simulink model "MotorControlLibNEWFixedP_FULL19b"  (R2020b)
settings: Solver=FixedStepDiscrete  StartTime=0.0  StopTime=100  FixedStep=Ts  RelTol=1e-3
values from neighbouring files (symbols this model uses):
  Ki_Iab_EMFobs = 1600.0    [MotorControl.sldd]
  Kp_Iab_EMFobs = 0.255    [MotorControl.sldd]
  p = 8/2    (= 4)    [MotorControlLibData.m]    (also in local_pmsm_torque_control_data.m = 8)
  Ts = 250.0e-06    (= 0.00025)    [MotorControlLibData.m]    (also in local_pmsm_torque_control_data.m = 5e-06)
undefined symbols (not defined in the file or in its folder): BrkPoints, CuttOffFreq_c, d_q_Voltage_Limiter_max, d_q_Voltage_Limiter_sat_neg, d_q_Voltage_Limiter_sat_pos, DiscIntNeverNeededParam, Down, dSoll, EMFobsLdGain, EMFobsRS, Ki_dAxis, Ki_qAxis, Kp_dAxis, Kp_qAxis, MaxBckEMFVol_sat_neg, MaxBckEMFVol_sat_pos, NumBits1, NumBits2, pwmTableData, qSoll, Slope1, Slope2, TqToIqConst, TsIntern, Up
libraries: simulink x13, pid_lib x6, eePwmGenerator x3, simulink_extras x2
(part 2 of 3)

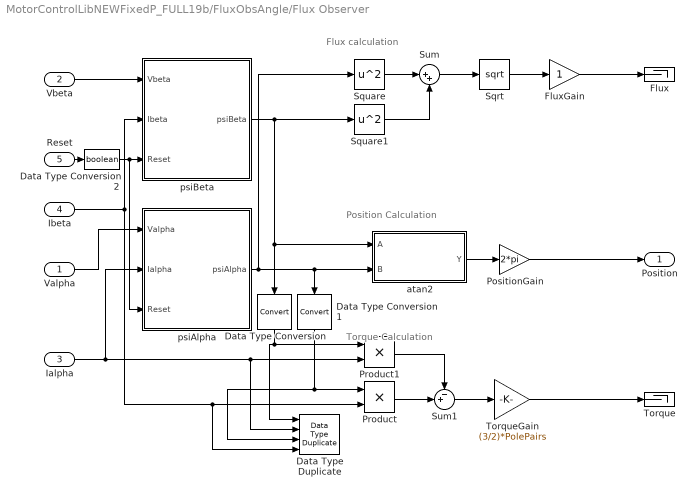
== system MotorControlLibNEWFixedP_FULL19b/FluxObsAngle/Flux Observer ==
  note: Torque Calculation
  note: Position Calculation
  note: Flux calculation
  Valpha : Inport  SampleTime=BlockSampleTime
  Vbeta : Inport  Port=2  SampleTime=BlockSampleTime
  Ialpha : Inport  Port=3  SampleTime=BlockSampleTime
  Ibeta : Inport  Port=4  SampleTime=BlockSampleTime
  Reset : Inport  Port=5  SampleTime=BlockSampleTime
  Data Type Duplicate : DataTypeDuplicate  NumInputPorts=4
  Data Type Conversion : DataTypeConversion  RndMeth=Simplest
  Data Type Conversion1 : DataTypeConversion  RndMeth=Simplest
  Data Type Conversion2 : DataTypeConversion  OutDataTypeStr=boolean  RndMeth=Simplest
  Flux : Terminator
  FluxGain : Gain  OutDataTypeStr=FluxDatatype  RndMeth=Simplest
  PositionGain : Gain  Gain=2*pi  OutDataTypeStr=PositionDatatype  RndMeth=Simplest
  Product : Product  RndMeth=Simplest  OutDataTypeStr=Inherit: Same as first input
  Product1 : Product  RndMeth=Simplest  OutDataTypeStr=Inherit: Same as first input
  Sqrt : Sqrt  RndMeth=Simplest  IntermediateResultsDataTypeStr=Inherit: Inherit from input  SaturateOnIntegerOverflow=on
  Square : Math  Operator=square  RndMeth=Simplest  SaturateOnIntegerOverflow=on
  Square1 : Math  Operator=square  RndMeth=Simplest  SaturateOnIntegerOverflow=on
  Sum : Sum  Inputs=|++
  Sum1 : Sum  Inputs=-+|
  Torque : Terminator
  TorqueGain : Gain  Gain=(3/2)*PolePairs  OutDataTypeStr=TorqueDatatype
  atan2 : Subsystem  TreatAsAtomicUnit=on  mask(atan2){outputUnit=PerUnit}
      mask prompts: outputUnit "Output unit:"
      mask help:
      | Compute the four-quadrant arctangent for two real numbers.
      |
      | The output datatype is identical to the inputs.
      |
      | The block output ranges from -pi to +pi (Radians) or 0 to 1 (PerUnit).
      mask Help: eval('mcb.internal.helpview(''atantwo'')')
      mask TypeOptions outputUnit: Radians | PerUnit
      mask Callback outputUnit: set_param([gcb, '/a16'],'AlgorithmParameterValue1',get_param(gcb,'outputUnit'))
      mask DialogControl Container7 Prompt: Parameters
      mask Display:
      | color('black');
      | port_label('input',1, 'A');
      | port_label('input',2, 'B');,
      | port_label('output',1, '\theta', 'interpreter', 'tex');
      | fprintf('atan2');
  psiAlpha : Subsystem
  psiBeta : Subsystem
  Position : Outport
  wires:
  Valpha/1 -> psiAlpha/1(Valpha)
  Ibeta/1 -> psiBeta/2(Ibeta), Data Type Duplicate/4, Product/2
  Vbeta/1 -> psiBeta/1(Vbeta)
  Reset/1 -> Data Type Conversion2/1
  TorqueGain/1 -> Torque/1
  Product/1 -> Sum1/2
  psiBeta/1(psiBeta) -> Square1/1, atan2/1(A), Data Type Conversion/1
  psiAlpha/1(psiAlpha) -> atan2/2(B), Data Type Conversion1/1, Square/1
  Ialpha/1 -> psiAlpha/2(Ialpha), Data Type Duplicate/2, Product1/2
  Product1/1 -> Sum1/1
  Sum1/1 -> TorqueGain/1
  FluxGain/1 -> Flux/1
  Square/1 -> Sum/1
  Sum/1 -> Sqrt/1
  Square1/1 -> Sum/2
  Sqrt/1 -> FluxGain/1
  PositionGain/1 -> Position/1
  atan2/1(Y) -> PositionGain/1
  Data Type Conversion/1 -> Data Type Duplicate/1, Product1/1
  Data Type Conversion1/1 -> Data Type Duplicate/3, Product/1
  Data Type Conversion2/1 -> psiAlpha/3(Reset), psiBeta/3(Reset)

== system MotorControlLibNEWFixedP_FULL19b/Inverse Park Transform/Switch_Axis ==
  A : Inport
  B : Inport  Port=2
  D_axis_aligned : Mux  Inputs=2
  Demux : Demux  Outputs=2
  Offset : Constant  Value=0  OutDataTypeStr=uint16  SampleTime=-1
  Q_axis_aligned : Mux  Inputs=2
  Switch : Switch  Criteria=u2 > Threshold  Threshold=1  RndMeth=Simplest  ZeroCross=off
  Unary_Minus : UnaryMinus
  Alpha : Outport  VectorParamsAs1DForOutWhenUnconnected=off
  Beta : Outport  Port=2  VectorParamsAs1DForOutWhenUnconnected=off
  wires:
  A/1 -> D_axis_aligned/1, Unary_Minus/1
  Unary_Minus/1 -> Q_axis_aligned/2
  Demux/2 -> Beta/1
  Switch/1 -> Demux/1
  B/1 -> D_axis_aligned/2, Q_axis_aligned/1
  Demux/1 -> Alpha/1
  Offset/1 -> Switch/2
  Q_axis_aligned/1 -> Switch/1
  D_axis_aligned/1 -> Switch/3

== system MotorControlLibNEWFixedP_FULL19b/PI_Controller/disable integrator on start up ==
  Add2 : Sum
  Compare To Constant : simulink/Logic and Bit Operations/Compare To Constant  relop=<  const=1500  OutDataTypeStr=boolean
  Constant8 : Constant  OutDataTypeStr=uint8
  Unit Delay : UnitDelay  SampleTime=-1  HasFrameUpgradeWarning=on
  time out : Outport
  wires:
  Add2/1 -> Unit Delay/1, Compare To Constant/1
  Constant8/1 -> Add2/1
  Compare To Constant/1 -> time out/1
  Unit Delay/1 -> Add2/2

== system MotorControlLibNEWFixedP_FULL19b/PWM Output/Inverse Clarke Transform ==
  In1 : Inport
  In2 : Inport  Port=2
  Data Type Duplicate : DataTypeDuplicate
  add_b : Sum  Inputs=-+  RndMeth=Simplest  OutDataTypeStr=Inherit: Same as first input
  add_c : Sum  Inputs=--  RndMeth=Simplest  OutDataTypeStr=Inherit: Same as first input
  one_by_two : Gain  Gain=1/2  RndMeth=Simplest  OutDataTypeStr=Inherit: Same as input
  sqrt3_by_two : Gain  Gain=sqrt(3)/2  RndMeth=Simplest  OutDataTypeStr=Inherit: Same as input
  a : Outport  VectorParamsAs1DForOutWhenUnconnected=off
  b : Outport  Port=2  VectorParamsAs1DForOutWhenUnconnected=off
  c : Outport  Port=3  VectorParamsAs1DForOutWhenUnconnected=off
  wires:
  add_c/1 -> c/1
  sqrt3_by_two/1 -> add_c/2, add_b/2
  In1/1 -> one_by_two/1, Data Type Duplicate/1, a/1
  one_by_two/1 -> add_b/1, add_c/1
  In2/1 -> sqrt3_by_two/1, Data Type Duplicate/2
  add_b/1 -> b/1

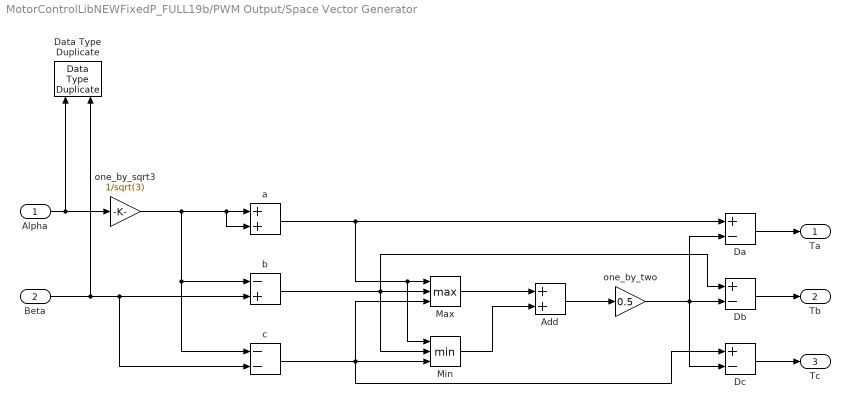
== system MotorControlLibNEWFixedP_FULL19b/PWM Output/Space Vector Generator ==
  Alpha : Inport
  Beta : Inport  Port=2
  Add : Sum  RndMeth=Simplest  OutDataTypeStr=Inherit: Same as first input
  Da : Sum  Inputs=+-  RndMeth=Simplest  OutDataTypeStr=Inherit: Same as first input
  Data Type Duplicate : DataTypeDuplicate
  Db : Sum  Inputs=+-  RndMeth=Simplest  OutDataTypeStr=Inherit: Same as first input
  Dc : Sum  Inputs=+-  RndMeth=Simplest  OutDataTypeStr=Inherit: Same as first input
  Max : MinMax  Function=max  Inputs=3  RndMeth=Simplest
  Min : MinMax  Inputs=3  RndMeth=Simplest
  a : Sum  RndMeth=Simplest  OutDataTypeStr=Inherit: Same as first input
  b : Sum  Inputs=-+  RndMeth=Simplest  OutDataTypeStr=Inherit: Same as first input
  c : Sum  Inputs=--  RndMeth=Simplest  OutDataTypeStr=Inherit: Same as first input
  one_by_sqrt3 : Gain  Gain=1/sqrt(3)  RndMeth=Simplest  OutDataTypeStr=Inherit: Same as input  ParamDataTypeStr=Inherit: Same as input
  one_by_two : Gain  Gain=0.5  RndMeth=Simplest  OutDataTypeStr=Inherit: Same as input  ParamDataTypeStr=Inherit: Same as input
  Ta : Outport  VectorParamsAs1DForOutWhenUnconnected=off
  Tb : Outport  Port=2  VectorParamsAs1DForOutWhenUnconnected=off
  Tc : Outport  Port=3  VectorParamsAs1DForOutWhenUnconnected=off
  wires:
  Db/1 -> Tb/1
  Dc/1 -> Tc/1
  Da/1 -> Ta/1
  a/1 -> Max/1, Min/1, Da/1
  Max/1 -> Add/1
  one_by_two/1 -> Da/2, Db/2, Dc/2
  Add/1 -> one_by_two/1
  Min/1 -> Add/2
  Alpha/1 -> Data Type Duplicate/1, one_by_sqrt3/1
  one_by_sqrt3/1 -> a/1, a/2, b/1, c/1
  Beta/1 -> c/2, b/2, Data Type Duplicate/2
  b/1 -> Max/2, Min/2, Db/1
  c/1 -> Min/3, Dc/1, Max/3

== system MotorControlLibNEWFixedP_FULL19b/Park Transform/Switch_Axis ==
  d : Inport
  q : Inport  Port=2
  D_axis_aligned : Mux  Inputs=2
  Demux : Demux  Outputs=2
  Offset : Constant  Value=0  OutDataTypeStr=uint16  SampleTime=-1
  Q_axis_aligned : Mux  Inputs=2
  Switch : Switch  Criteria=u2 > Threshold  Threshold=1  RndMeth=Simplest  ZeroCross=off
  Unary_Minus : UnaryMinus
  d_axis : Outport  VectorParamsAs1DForOutWhenUnconnected=off
  q_axis : Outport  Port=2  VectorParamsAs1DForOutWhenUnconnected=off
  wires:
  D_axis_aligned/1 -> Switch/3
  Q_axis_aligned/1 -> Switch/1
  d/1 -> D_axis_aligned/1, Q_axis_aligned/2
  Offset/1 -> Switch/2
  Demux/1 -> d_axis/1
  Unary_Minus/1 -> Q_axis_aligned/1
  q/1 -> D_axis_aligned/2, Unary_Minus/1
  Switch/1 -> Demux/1
  Demux/2 -> q_axis/1

== system MotorControlLibNEWFixedP_FULL19b/Position observer/Atan2 ==
  In1 : Inport
  In2 : Inport  Port=2
  Atan2 : Trigonometry  Operator=atan2  ApproximationMethod=CORDIC  NumberOfIterations=6
  Data Type Conversion5 : DataTypeConversion
  Data Type Conversion6 : DataTypeConversion  OutDataTypeStr=single
  Data Type Conversion7 : DataTypeConversion  OutDataTypeStr=single
  Out1 : Outport
  wires:
  Atan2/1 -> Data Type Conversion5/1
  In1/1 -> Data Type Conversion6/1
  Data Type Conversion6/1 -> Atan2/1
  Data Type Conversion7/1 -> Atan2/2
  In2/1 -> Data Type Conversion7/1
  Data Type Conversion5/1 -> Out1/1

== system MotorControlLibNEWFixedP_FULL19b/Position observer/EMF Observer Ia ==
  Iab : Inport
  Vab : Inport  Port=2
  filtered emf : Inport  Port=3
  reset : Inport  Port=4
  Add6 : Sum  Inputs=-+  InputSameDT=on
  DC Motor Model : Subsystem  TreatAsAtomicUnit=on  SystemSampleTime=Ts
  PI Controller : Subsystem
  Rate Transition{,1..3} (4 alike) : RateTransition  Integrity=off
  Unit Delay : UnitDelay  SampleTime=-1  HasFrameUpgradeWarning=on
  BackEMFest : Outport
  wires:
  Iab/1 -> Add6/1
  DC Motor Model/1(i_integrated_en8) -> Rate Transition/1
  Vab/1 -> Rate Transition1/1
  Rate Transition/1 -> Add6/2  "Iest"
  Rate Transition1/1 -> DC Motor Model/2(In2)
  Rate Transition2/1 -> DC Motor Model/1(Sig_Emfobs_PI_out)
  PI Controller/1(Sig_Emfobs_PI_out) -> Unit Delay/1, BackEMFest/1  "BackEMF est"
  Add6/1 -> PI Controller/1(Sig_Emfobs_errorSum_m)  "Sig_Emfobs_errorSum_m"
  filtered emf/1 -> Rate Transition3/1
  Rate Transition3/1 -> DC Motor Model/3(In3)
  Unit Delay/1 -> Rate Transition2/1
  reset/1 -> PI Controller/2(reset)

== system MotorControlLibNEWFixedP_FULL19b/Position observer/EMF Observer Ia1 ==
  Iab : Inport
  Vab : Inport  Port=2
  DC Motor Model : Subsystem
  PI Controller : Subsystem
  Rate Transition : RateTransition
  Rate Transition1 : RateTransition
  Rate Transition2 : RateTransition
  Unit Delay : UnitDelay  SampleTime=-1  HasFrameUpgradeWarning=on
  Iestimated : Outport
  IestNEW : Outport  Port=2
  wires:
  DC Motor Model/1(Out1) -> Rate Transition/1
  Vab/1 -> Rate Transition1/1
  Rate Transition/1 -> PI Controller/2(In2), IestNEW/1
  Rate Transition1/1 -> DC Motor Model/2(In2)
  Rate Transition2/1 -> DC Motor Model/1(In1)
  PI Controller/1(Out1) -> Iestimated/1, Unit Delay/1
  Iab/1 -> PI Controller/1(In1)
  Unit Delay/1 -> Rate Transition2/1

== system MotorControlLibNEWFixedP_FULL19b/Position observer/EMF Observer Ia2 ==
  Iab : Inport
  Vab : Inport  Port=2
  filtered emf : Inport  Port=3
  reset : Inport  Port=4
  Add6 : Sum  Inputs=-+  InputSameDT=on
  DC Motor Model : Subsystem  TreatAsAtomicUnit=on  SystemSampleTime=Ts
  Data Type Conversion : DataTypeConversion
  PI Controller : Subsystem  TreatAsAtomicUnit=on
  Rate Transition{,1..3} (4 alike) : RateTransition  Integrity=off
  Unit Delay : UnitDelay  SampleTime=-1  HasFrameUpgradeWarning=on
  BackEMFest : Outport
  wires:
  PI Controller/1(Sig_Emfobs_PI_out) -> Unit Delay/1, BackEMFest/1
  Add6/1 -> PI Controller/1(Sig_Emfobs_errorSum_m)
  Rate Transition2/1 -> DC Motor Model/1(Sig_Emfobs_PI_out)
  Rate Transition1/1 -> DC Motor Model/2(In2)
  Rate Transition/1 -> Add6/2
  Vab/1 -> Rate Transition1/1
  DC Motor Model/1(i_integrated_en8) -> Rate Transition/1
  Iab/1 -> Data Type Conversion/1
  Data Type Conversion/1 -> Add6/1
  filtered emf/1 -> Rate Transition3/1
  Rate Transition3/1 -> DC Motor Model/3(Sig_Emfobs_PI_out1)
  Unit Delay/1 -> Rate Transition2/1
  reset/1 -> PI Controller/2(reset)

== system MotorControlLibNEWFixedP_FULL19b/Position observer/Low pass filter ==
  note: Integrator
  note: d/dt(i)
  In1 : Inport
  Add2 : Sum  Inputs=+-
  Constant : Constant  Value=Value  OutDataTypeStr=uint16
  Delay : Delay  DelayLength=1  InitialCondition=0
  Gain : Gain  Gain=Gain  ParamDataTypeStr=fixdt(1,16,2^-16,0)  OutDataTypeStr=fixdt(1,16,2^-14,0)  SaturateOnIntegerOverflow=on
  Product1 : Product  OutDataTypeStr=fixdt(1,16,2^-6,0)
  Sum : Sum  Inputs=|++  OutDataTypeStr=Inherit: Same as first input
  Unit Delay : UnitDelay  SampleTime=-1  HasFrameUpgradeWarning=on
  Output : Outport
  wires:
  Constant/1 -> Product1/2
  In1/1 -> Add2/1
  Add2/1 -> Gain/1
  Product1/1 -> Output/1, Unit Delay/1
  Gain/1 -> Sum/1
  Delay/1 -> Sum/2
  Sum/1 -> Delay/1, Product1/1
  Unit Delay/1 -> Add2/2

== system MotorControlLibNEWFixedP_FULL19b/Position observer/Low pass filter1 ==
  note: d/dt(i)
  note: Integrator
  In1 : Inport
  Add2 : Sum  Inputs=+-
  Constant : Constant  Value=Value  OutDataTypeStr=uint16
  Delay : Delay  DelayLength=1  InitialCondition=0
  Gain : Gain  Gain=Gain  ParamDataTypeStr=fixdt(1,16,2^-16,0)  OutDataTypeStr=fixdt(1,16,2^-14,0)  SaturateOnIntegerOverflow=on
  Product1 : Product  OutDataTypeStr=fixdt(1,16,2^-6,0)
  Sum : Sum  Inputs=|++  OutDataTypeStr=Inherit: Same as first input
  Unit Delay : UnitDelay  SampleTime=-1  HasFrameUpgradeWarning=on
  Output : Outport
  wires:
  Unit Delay/1 -> Add2/2
  Sum/1 -> Product1/1, Delay/1
  Delay/1 -> Sum/2
  Gain/1 -> Sum/1
  Product1/1 -> Unit Delay/1, Output/1
  Add2/1 -> Gain/1
  In1/1 -> Add2/1
  Constant/1 -> Product1/2

== system MotorControlLibNEWFixedP_FULL19b/Position observer/Low pass filter2 ==
  note: Integrator
  note: d/dt(i)
  In1 : Inport
  Add2 : Sum  Inputs=+-
  Constant : Constant  Value=Value  OutDataTypeStr=uint16
  Delay : Delay  DelayLength=1  InitialCondition=0
  Gain : Gain  Gain=Gain  ParamDataTypeStr=fixdt(1,16,2^-16,0)  OutDataTypeStr=fixdt(1,16,2^-14,0)  SaturateOnIntegerOverflow=on
  Product1 : Product  OutDataTypeStr=fixdt(1,16,2^-6,0)
  Sum : Sum  Inputs=|++  OutDataTypeStr=Inherit: Same as first input
  Unit Delay : UnitDelay  SampleTime=-1  HasFrameUpgradeWarning=on
  Output : Outport
  wires:
  Constant/1 -> Product1/2
  In1/1 -> Add2/1
  Add2/1 -> Gain/1
  Product1/1 -> Output/1, Unit Delay/1
  Gain/1 -> Sum/1
  Delay/1 -> Sum/2
  Sum/1 -> Delay/1, Product1/1
  Unit Delay/1 -> Add2/2

== system MotorControlLibNEWFixedP_FULL19b/Position observer/Low pass filter3 ==
  note: d/dt(i)
  note: Integrator
  In1 : Inport
  Add2 : Sum  Inputs=+-
  Constant : Constant  Value=Value  OutDataTypeStr=uint16
  Delay : Delay  DelayLength=1  InitialCondition=0
  Gain : Gain  Gain=Gain  ParamDataTypeStr=fixdt(1,16,2^-16,0)  OutDataTypeStr=fixdt(1,16,2^-14,0)  SaturateOnIntegerOverflow=on
  Product1 : Product  OutDataTypeStr=fixdt(1,16,2^-6,0)
  Sum : Sum  Inputs=|++  OutDataTypeStr=Inherit: Same as first input
  Unit Delay : UnitDelay  SampleTime=-1  HasFrameUpgradeWarning=on
  Output : Outport
  wires:
  Unit Delay/1 -> Add2/2
  Sum/1 -> Product1/1, Delay/1
  Delay/1 -> Sum/2
  Gain/1 -> Sum/1
  Product1/1 -> Unit Delay/1, Output/1
  Add2/1 -> Gain/1
  In1/1 -> Add2/1
  Constant/1 -> Product1/2

== system MotorControlLibNEWFixedP_FULL19b/Position observer fixed point/Atan2 ==
  In1 : Inport
  In2 : Inport  Port=2
  Atan2 : Trigonometry  Operator=atan2  ApproximationMethod=CORDIC  NumberOfIterations=6
  Data Type Conversion5 : DataTypeConversion
  Data Type Conversion6 : DataTypeConversion  OutDataTypeStr=single
  Data Type Conversion7 : DataTypeConversion  OutDataTypeStr=single
  Out1 : Outport
  wires:
  Atan2/1 -> Data Type Conversion5/1
  In1/1 -> Data Type Conversion6/1
  Data Type Conversion6/1 -> Atan2/1
  Data Type Conversion7/1 -> Atan2/2
  In2/1 -> Data Type Conversion7/1
  Data Type Conversion5/1 -> Out1/1

== system MotorControlLibNEWFixedP_FULL19b/Position observer fixed point/EMF Observer Ia ==
  Iab : Inport
  Vab : Inport  Port=2
  filtered emf : Inport  Port=3
  reset : Inport  Port=4
  Add6 : Sum  Inputs=-+  InputSameDT=on
  DC Motor Model : Subsystem  TreatAsAtomicUnit=on  SystemSampleTime=Ts
  PI Controller : Subsystem
  Rate Transition{,1..3} (4 alike) : RateTransition  Integrity=off
  Unit Delay : UnitDelay  SampleTime=-1  HasFrameUpgradeWarning=on
  BackEMFest : Outport
  wires:
  Iab/1 -> Add6/1
  DC Motor Model/1(i_integrated_en8) -> Rate Transition/1
  Vab/1 -> Rate Transition1/1
  Rate Transition/1 -> Add6/2  "Iest"
  Rate Transition1/1 -> DC Motor Model/2(In2)
  Rate Transition2/1 -> DC Motor Model/1(Sig_Emfobs_PI_out)
  PI Controller/1(Sig_Emfobs_PI_out) -> Unit Delay/1, BackEMFest/1  "BackEMF est"
  Add6/1 -> PI Controller/1(Sig_Emfobs_errorSum_m)  "Sig_Emfobs_errorSum_m"
  filtered emf/1 -> Rate Transition3/1
  Rate Transition3/1 -> DC Motor Model/3(In3)
  Unit Delay/1 -> Rate Transition2/1
  reset/1 -> PI Controller/2(reset)

== system MotorControlLibNEWFixedP_FULL19b/Position observer fixed point/EMF Observer Ia1 ==
  Iab : Inport
  Vab : Inport  Port=2
  DC Motor Model : Subsystem
  PI Controller : Subsystem
  Rate Transition : RateTransition
  Rate Transition1 : RateTransition
  Rate Transition2 : RateTransition
  Unit Delay : UnitDelay  SampleTime=-1  HasFrameUpgradeWarning=on
  Iestimated : Outport
  IestNEW : Outport  Port=2
  wires:
  DC Motor Model/1(Out1) -> Rate Transition/1
  Vab/1 -> Rate Transition1/1
  Rate Transition/1 -> PI Controller/2(In2), IestNEW/1
  Rate Transition1/1 -> DC Motor Model/2(In2)
  Rate Transition2/1 -> DC Motor Model/1(In1)
  PI Controller/1(Out1) -> Iestimated/1, Unit Delay/1
  Iab/1 -> PI Controller/1(In1)
  Unit Delay/1 -> Rate Transition2/1

== system MotorControlLibNEWFixedP_FULL19b/Position observer fixed point/EMF Observer Ia2 ==
  Iab : Inport
  Vab : Inport  Port=2
  filtered emf : Inport  Port=3
  reset : Inport  Port=4
  Add6 : Sum  Inputs=-+  InputSameDT=on
  DC Motor Model : Subsystem  TreatAsAtomicUnit=on  SystemSampleTime=Ts
  Data Type Conversion : DataTypeConversion
  PI Controller : Subsystem  TreatAsAtomicUnit=on
  Rate Transition{,1..3} (4 alike) : RateTransition  Integrity=off
  Unit Delay : UnitDelay  SampleTime=-1  HasFrameUpgradeWarning=on
  BackEMFest : Outport
  wires:
  PI Controller/1(Sig_Emfobs_PI_out) -> Unit Delay/1, BackEMFest/1
  Add6/1 -> PI Controller/1(Sig_Emfobs_errorSum_m)
  Rate Transition2/1 -> DC Motor Model/1(Sig_Emfobs_PI_out)
  Rate Transition1/1 -> DC Motor Model/2(In2)
  Rate Transition/1 -> Add6/2
  Vab/1 -> Rate Transition1/1
  DC Motor Model/1(i_integrated_en8) -> Rate Transition/1
  Iab/1 -> Data Type Conversion/1
  Data Type Conversion/1 -> Add6/1
  filtered emf/1 -> Rate Transition3/1
  Rate Transition3/1 -> DC Motor Model/3(Sig_Emfobs_PI_out1)
  Unit Delay/1 -> Rate Transition2/1
  reset/1 -> PI Controller/2(reset)

== system MotorControlLibNEWFixedP_FULL19b/Position observer fixed point/Low pass filter ==
  note: Integrator
  note: d/dt(i)
  In1 : Inport
  Add2 : Sum  Inputs=+-
  Constant : Constant  Value=Value  OutDataTypeStr=uint16
  Delay : Delay  DelayLength=1  InitialCondition=0
  Gain : Gain  Gain=Gain  ParamDataTypeStr=fixdt(1,16,2^-16,0)  OutDataTypeStr=fixdt(1,16,2^-14,0)  SaturateOnIntegerOverflow=on
  Product1 : Product  OutDataTypeStr=fixdt(1,16,2^-6,0)
  Sum : Sum  Inputs=|++  OutDataTypeStr=Inherit: Same as first input
  Unit Delay : UnitDelay  SampleTime=-1  HasFrameUpgradeWarning=on
  Output : Outport
  wires:
  Constant/1 -> Product1/2
  In1/1 -> Add2/1
  Add2/1 -> Gain/1
  Product1/1 -> Output/1, Unit Delay/1
  Gain/1 -> Sum/1
  Delay/1 -> Sum/2
  Sum/1 -> Delay/1, Product1/1
  Unit Delay/1 -> Add2/2

== system MotorControlLibNEWFixedP_FULL19b/Position observer fixed point/Low pass filter1 ==
  note: d/dt(i)
  note: Integrator
  In1 : Inport
  Add2 : Sum  Inputs=+-
  Constant : Constant  Value=Value  OutDataTypeStr=uint16
  Delay : Delay  DelayLength=1  InitialCondition=0
  Gain : Gain  Gain=Gain  ParamDataTypeStr=fixdt(1,16,2^-16,0)  OutDataTypeStr=fixdt(1,16,2^-14,0)  SaturateOnIntegerOverflow=on
  Product1 : Product  OutDataTypeStr=fixdt(1,16,2^-6,0)
  Sum : Sum  Inputs=|++  OutDataTypeStr=Inherit: Same as first input
  Unit Delay : UnitDelay  SampleTime=-1  HasFrameUpgradeWarning=on
  Output : Outport
  wires:
  Unit Delay/1 -> Add2/2
  Sum/1 -> Product1/1, Delay/1
  Delay/1 -> Sum/2
  Gain/1 -> Sum/1
  Product1/1 -> Unit Delay/1, Output/1
  Add2/1 -> Gain/1
  In1/1 -> Add2/1
  Constant/1 -> Product1/2

== system MotorControlLibNEWFixedP_FULL19b/Position observer fixed point/Low pass filter2 ==
  note: Integrator
  note: d/dt(i)
  In1 : Inport
  Add2 : Sum  Inputs=+-
  Constant : Constant  Value=Value  OutDataTypeStr=uint16
  Delay : Delay  DelayLength=1  InitialCondition=0
  Gain : Gain  Gain=Gain  ParamDataTypeStr=fixdt(1,16,2^-16,0)  OutDataTypeStr=fixdt(1,16,2^-14,0)  SaturateOnIntegerOverflow=on
  Product1 : Product  OutDataTypeStr=fixdt(1,16,2^-6,0)
  Sum : Sum  Inputs=|++  OutDataTypeStr=Inherit: Same as first input
  Unit Delay : UnitDelay  SampleTime=-1  HasFrameUpgradeWarning=on
  Output : Outport
  wires:
  Constant/1 -> Product1/2
  In1/1 -> Add2/1
  Add2/1 -> Gain/1
  Product1/1 -> Output/1, Unit Delay/1
  Gain/1 -> Sum/1
  Delay/1 -> Sum/2
  Sum/1 -> Delay/1, Product1/1
  Unit Delay/1 -> Add2/2

== system MotorControlLibNEWFixedP_FULL19b/Position observer fixed point/Low pass filter3 ==
  note: d/dt(i)
  note: Integrator
  In1 : Inport
  Add2 : Sum  Inputs=+-
  Constant : Constant  Value=Value  OutDataTypeStr=uint16
  Delay : Delay  DelayLength=1  InitialCondition=0
  Gain : Gain  Gain=Gain  ParamDataTypeStr=fixdt(1,16,2^-16,0)  OutDataTypeStr=fixdt(1,16,2^-14,0)  SaturateOnIntegerOverflow=on
  Product1 : Product  OutDataTypeStr=fixdt(1,16,2^-6,0)
  Sum : Sum  Inputs=|++  OutDataTypeStr=Inherit: Same as first input
  Unit Delay : UnitDelay  SampleTime=-1  HasFrameUpgradeWarning=on
  Output : Outport
  wires:
  Unit Delay/1 -> Add2/2
  Sum/1 -> Product1/1, Delay/1
  Delay/1 -> Sum/2
  Gain/1 -> Sum/1
  Product1/1 -> Unit Delay/1, Output/1
  Add2/1 -> Gain/1
  In1/1 -> Add2/1
  Constant/1 -> Product1/2

== system MotorControlLibNEWFixedP_FULL19b/Start up/Logic after motor is stoped ==
  In1 : Inport
  Compare To Zero : simulink/Logic and Bit Operations/Compare To Zero  relop===  OutDataTypeStr=boolean
  Detect Decrease : simulink/Logic and Bit Operations/Detect Decrease  vinit=0  OutDataTypeStr=boolean
  Enabled Subsystem : Subsystem  TreatAsAtomicUnit=on
  Enabled Subsystem1 : Subsystem  TreatAsAtomicUnit=on
  S-R Flip-Flop : simulink_extras/Flip Flops/S-R Flip-Flop  initial_condition=0
  S-R Flip-Flop1 : simulink_extras/Flip Flops/S-R Flip-Flop  initial_condition=0
  Terminator : Terminator
  Terminator1 : Terminator
  Unit Delay : UnitDelay  SampleTime=-1  HasFrameUpgradeWarning=on
  Unit Delay1 : UnitDelay  SampleTime=-1  HasFrameUpgradeWarning=on
  Out1 : Outport
  wires:
  Enabled Subsystem/1(Out1) -> S-R Flip-Flop1/1
  In1/1 -> Enabled Subsystem/1(In1), Compare To Zero/1
  S-R Flip-Flop/2 -> Terminator/1
  Enabled Subsystem1/1(Output) -> Out1/1, Unit Delay1/1
  S-R Flip-Flop/1 -> Enabled Subsystem/Enable
  S-R Flip-Flop1/1 -> Enabled Subsystem1/Enable, Unit Delay/1
  Unit Delay/1 -> S-R Flip-Flop/2
  Compare To Zero/1 -> S-R Flip-Flop/1
  S-R Flip-Flop1/2 -> Terminator1/1
  Unit Delay1/1 -> Detect Decrease/1
  Detect Decrease/1 -> S-R Flip-Flop1/2

== system MotorControlLibNEWFixedP_FULL19b/Start up/Simulate start up Theta ==
  note: Overflow danger
  In1 : Inport
  Abs : Abs
  Constant : Constant  Value=2*pi  OutDataTypeStr=fixdt(1,16,2^-8,0)
  Discrete-Time Integrator : DiscreteIntegrator  ExternalReset=rising  SampleTime=-1  OutDataTypeStr=fixdt(1,16,2^-8,0)  ICPrevOutput=DiscIntNeverNeededParam  ICPrevScaledInput=DiscIntNeverNeededParam
  Relational Operator : RelationalOperator  OutDataTypeStr=boolean  RndMeth=Simplest
  Unit Delay : UnitDelay  SampleTime=-1  HasFrameUpgradeWarning=on
  Out1 : Outport
  wires:
  Constant/1 -> Relational Operator/2
  Relational Operator/1 -> Unit Delay/1
  Unit Delay/1 -> Discrete-Time Integrator/2
  In1/1 -> Discrete-Time Integrator/1
  Discrete-Time Integrator/1 -> Out1/1, Abs/1
  Abs/1 -> Relational Operator/1

== system MotorControlLibNEWFixedP_FULL19b/CosSin/Sine-Cosine Lookup/Interpolation ==
  In1 : Inport
  In2 : Inport  Port=2
  Demux : Demux
  Product : Product  RndMeth=Simplest  OutDataTypeStr=Inherit: Same as first input
  Product1 : Product  RndMeth=Simplest  OutDataTypeStr=Inherit: Same as first input
  Sum3 : Sum  Inputs=|+-  RndMeth=Simplest  OutDataTypeStr=Inherit: Same as first input
  Sum4 : Sum  Inputs=|++  RndMeth=Simplest  OutDataTypeStr=Inherit: Same as first input
  Sum5 : Sum  Inputs=|+-  RndMeth=Simplest  OutDataTypeStr=Inherit: Same as first input
  Sum6 : Sum  Inputs=|++  RndMeth=Simplest  OutDataTypeStr=Inherit: Same as first input
  Out1 : Outport
  Out2 : Outport  Port=2
  wires:
  Sum4/1 -> Out1/1
  Sum6/1 -> Out2/1
  Demux/1 -> Sum3/1
  Sum5/1 -> Product1/1
  Demux/2 -> Sum3/2, Sum4/2
  In2/1 -> Product/2, Product1/2
  Product/1 -> Sum4/1
  Demux/4 -> Sum6/2, Sum5/2
  Product1/1 -> Sum6/1
  In1/1 -> Demux/1
  Sum3/1 -> Product/1
  Demux/3 -> Sum5/1

== system MotorControlLibNEWFixedP_FULL19b/CosSin/Sine-Cosine Lookup/WrapUp ==
  In1 : Inport
  Compare To Zero : simulink/Logic and Bit Operations/Compare To Zero  relop=<  OutDataTypeStr=boolean
  Data Type Conversion : DataTypeConversion  OutDataTypeStr=uint16  ConvertRealWorld=Stored Integer (SI)  RndMeth=Simplest
  If : If
  If Action Subsystem : Subsystem  TreatAsAtomicUnit=on
  If Action Subsystem1 : Subsystem  TreatAsAtomicUnit=on
  Merge : Merge
  convert_pu : Gain  Gain=1/(dlgSett.UpperSatLimit)  RndMeth=Simplest  OutDataTypeStr=Inherit: Same as input
  Out1 : Outport
  wires:
  In1/1 -> convert_pu/1
  If/1 -> If Action Subsystem/Action
  If/2 -> If Action Subsystem1/Action
  convert_pu/1 -> Compare To Zero/1, If Action Subsystem/1(In1), If Action Subsystem1/1(In1)
  If Action Subsystem/1(Out1) -> Merge/1
  If Action Subsystem1/1(Out1) -> Merge/2
  Compare To Zero/1 -> Data Type Conversion/1
  Data Type Conversion/1 -> If/1
  Merge/1 -> Out1/1

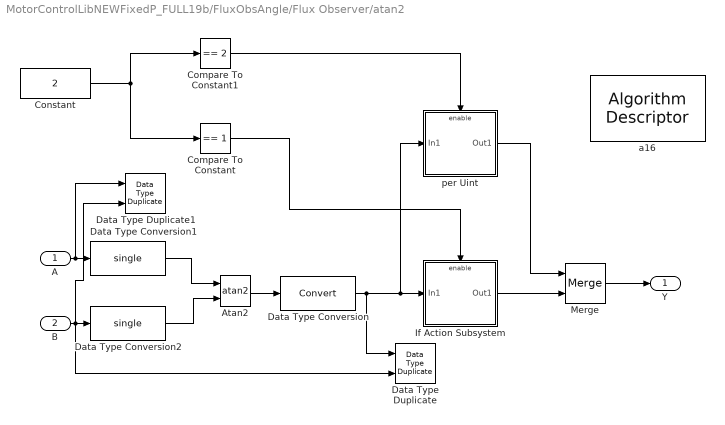
== system MotorControlLibNEWFixedP_FULL19b/FluxObsAngle/Flux Observer/atan2 ==
  A : Inport
  B : Inport  Port=2
  Atan2 : Trigonometry  Operator=atan2
  Compare To Constant : simulink/Logic and Bit Operations/Compare To Constant  relop===  const=1  OutDataTypeStr=boolean
  Compare To Constant1 : simulink/Logic and Bit Operations/Compare To Constant  relop===  const=2  OutDataTypeStr=boolean
  Constant : Constant  Value=2  OutDataTypeStr=uint16
  Data Type Duplicate : DataTypeDuplicate
  Data Type Duplicate1 : DataTypeDuplicate
  Data Type Conversion : DataTypeConversion
  Data Type Conversion1 : DataTypeConversion  OutDataTypeStr=single
  Data Type Conversion2 : DataTypeConversion  OutDataTypeStr=single
  If Action Subsystem : Subsystem  TreatAsAtomicUnit=on
  Merge : Merge
  a16 : AlgorithmDescriptor  AlgorithmName=trig_atan2  NumberOfInputs=2  InputBlockPath1=A  InputBlockPath2=B  ParameterBlockPath1=Constant  ParameterName1=Value  OutputBlockPath1=Y  OutputBlockPath2=Y2  NumberOfAlgorithmParameters=1  AlgorithmParameterName1=outputUnit  AlgorithmParameterValue1=PerUnit  AlgorithmParameterPrimary1=on
  per Uint : Subsystem  TreatAsAtomicUnit=on
  Y : Outport
  wires:
  Compare To Constant/1 -> If Action Subsystem/Enable
  Constant/1 -> Compare To Constant1/1, Compare To Constant/1
  Compare To Constant1/1 -> per Uint/Enable
  If Action Subsystem/1(Out1) -> Merge/2
  Atan2/1 -> Data Type Conversion/1
  per Uint/1(Out1) -> Merge/1
  Merge/1 -> Y/1
  A/1 -> Data Type Duplicate1/1, Data Type Conversion1/1
  B/1 -> Data Type Duplicate/2, Data Type Duplicate1/2, Data Type Conversion2/1
  Data Type Conversion1/1 -> Atan2/1
  Data Type Conversion2/1 -> Atan2/2
  Data Type Conversion/1 -> Data Type Duplicate/1, per Uint/1(In1), If Action Subsystem/1(In1)

== system MotorControlLibNEWFixedP_FULL19b/FluxObsAngle/Flux Observer/psiAlpha ==
  note: Integrator
  Valpha : Inport
  Ialpha : Inport  Port=2
  Reset : Inport  Port=3
  Constant : Constant  Value=1e-6  OutDataTypeStr=Inherit: Inherit via back propagation
  Data Type Duplicate : DataTypeDuplicate
  Data Type Propagation : simulink/Signal Attributes/Data Type Propagation  PropDataType=fixdt(1, 16)  IfRefDouble=double  IfRefSingle=single  IsSigned=IsSigned1 or IsSigned2  NumBitsBase=max([NumBits1 NumBits2])  NumBitsMult=1  NumBitsAdd=0  NumBitsAllowFinal=1:128  PropScalingMode=Obtain via best precision  PropScaling=2^-10  ValuesUsedBestPrec=[4 -4]  SlopeBase=min([Slope1 Slope2])  SlopeMult=1  SlopeAdd=0  BiasBase=Bias1  BiasMult=1  BiasAdd=0
      settings: SourceProductBaseCode=SL
  Delay : Delay  DelayLength=1  ExternalReset=Level
      settings: InputPortMap=u0,r5
  Gain : Gain  Gain=fi(BlockSampleTime(1),0,16)  ParamDataTypeStr=Inherit: Inherit from 'Gain'  OutDataTypeStr=Inherit: Inherit via back propagation
  Scaling : Subsystem
  Sum : Sum  Inputs=|++  RndMeth=Simplest  OutDataTypeStr=Inherit: Same as first input
  Sum1 : Sum  Inputs=|+-  RndMeth=Simplest  OutDataTypeStr=Inherit: Same as first input
  Sum3 : Sum  Inputs=|+-  RndMeth=Simplest  OutDataTypeStr=Inherit: Same as first input
  Switch : Switch  Criteria=u2 > Threshold
  psiAlpha : Outport
  wires:
  Sum/1 -> Sum1/1, Delay/1
  Valpha/1 -> Scaling/1("Valpha ")
  Ialpha/1 -> Scaling/2(Ialpha)
  Scaling/1(ValphaScaled) -> Sum3/1
  Scaling/2(IalphaScaled*R) -> Sum3/2
  Delay/1 -> Sum/2
  Sum3/1 -> Data Type Propagation/2, Data Type Propagation/1, Gain/1
  Gain/1 -> Data Type Propagation/3, Sum/1
  Sum1/1 -> Switch/3, Data Type Duplicate/1
  Scaling/3(IalphaScaled*L) -> Sum1/2
  Reset/1 -> Delay/2, Switch/2
  Constant/1 -> Data Type Duplicate/2, Switch/1
  Switch/1 -> psiAlpha/1

== system MotorControlLibNEWFixedP_FULL19b/FluxObsAngle/Flux Observer/psiBeta ==
  note: Integrator
  Vbeta : Inport
  Ibeta : Inport  Port=2
  Reset : Inport  Port=3
  Constant : Constant  Value=0  OutDataTypeStr=Inherit: Inherit via back propagation
  Data Type Duplicate : DataTypeDuplicate
  Data Type Propagation : simulink/Signal Attributes/Data Type Propagation  PropDataType=fixdt(1, 16)  IfRefDouble=double  IfRefSingle=single  IsSigned=IsSigned1 or IsSigned2  NumBitsBase=max([NumBits1 NumBits2])  NumBitsMult=1  NumBitsAdd=0  NumBitsAllowFinal=1:128  PropScalingMode=Obtain via best precision  PropScaling=2^-10  ValuesUsedBestPrec=[4 -4]  SlopeBase=min([Slope1 Slope2])  SlopeMult=1  SlopeAdd=0  BiasBase=Bias1  BiasMult=1  BiasAdd=0
      settings: SourceProductBaseCode=SL
  Delay : Delay  DelayLength=1  InitialCondition=0  ExternalReset=Level
      settings: InputPortMap=u0,r5
  Gain : Gain  Gain=fi(BlockSampleTime(1),0,16)  ParamDataTypeStr=Inherit: Inherit from 'Gain'  OutDataTypeStr=Inherit: Inherit via back propagation
  Scaling : Subsystem
  Sum : Sum  Inputs=|++  OutDataTypeStr=Inherit: Same as first input
  Sum1 : Sum  Inputs=|+-  RndMeth=Simplest  OutDataTypeStr=Inherit: Same as first input
  Sum3 : Sum  Inputs=|+-  RndMeth=Simplest  OutDataTypeStr=Inherit: Same as first input
  Switch : Switch  Criteria=u2 > Threshold
  psiBeta : Outport
  wires:
  Sum/1 -> Sum1/1, Delay/1
  Vbeta/1 -> Scaling/1(Vbeta)
  Ibeta/1 -> Scaling/2(Ibeta)
  Scaling/2(IbetaScaled*R) -> Sum3/2
  Scaling/1(VbetaScaled) -> Sum3/1
  Delay/1 -> Sum/2
  Sum3/1 -> Data Type Propagation/2, Data Type Propagation/1, Gain/1
  Gain/1 -> Data Type Propagation/3, Sum/1
  Reset/1 -> Delay/2, Switch/2
  Scaling/3(IbetaScaled*L) -> Sum1/2
  Sum1/1 -> Data Type Duplicate/1, Switch/3
  Switch/1 -> psiBeta/1
  Constant/1 -> Data Type Duplicate/2, Switch/1

== system MotorControlLibNEWFixedP_FULL19b/Position observer/EMF Observer Ia/DC Motor Model ==
  note: d/dt(i)
  note: Integrator
  Sig_Emfobs_PI_out : Inport
  In2 : Inport  Port=2
  In3 : Inport  Port=3
  Add5 : Sum  Inputs=-+--  OutDataTypeStr=Inherit: Same as first input
  Data Type Conversion : DataTypeConversion
  Delay : Delay  DelayLength=1  InitialCondition=0  StateName=UnitDelayIntegratorPosObs
  Gain : Gain  Gain=TsIntern  ParamDataTypeStr=Inherit: Inherit from 'Gain'  OutMin=-100  OutMax=+100  OutDataTypeStr=single  SaturateOnIntegerOverflow=on
  Inductance : Gain  Gain=Ld  OutDataTypeStr=single
  Resistance : Gain  Gain=Rs  OutDataTypeStr=Inherit: Inherit via back propagation
  Sum : Sum  Inputs=|++  OutDataTypeStr=Inherit: Same as first input
  Unit Delay : UnitDelay  SampleTime=-1  HasFrameUpgradeWarning=on
  i_integrated_en8 : Outport
  wires:
  Unit Delay/1 -> Inductance/1
  Gain/1 -> Sum/1  "di_dt_times_Ts_En8"
  Sum/1 -> Delay/1, Data Type Conversion/1, Resistance/1  "i_integrated_en4"
  In2/1 -> Add5/2
  Resistance/1 -> Add5/1  "i_integrated_times_Rs_en8"
  Delay/1 -> Sum/2
  Sig_Emfobs_PI_out/1 -> Add5/3
  Add5/1 -> Unit Delay/1  "Va_all_16En4"
  Inductance/1 -> Gain/1  "di_dt_E9"
  Data Type Conversion/1 -> i_integrated_en8/1
  In3/1 -> Add5/4

== system MotorControlLibNEWFixedP_FULL19b/Position observer/EMF Observer Ia/PI Controller ==
  Sig_Emfobs_errorSum_m : Inport
  reset : Inport  Port=2
  Abs : Abs
  Add1 : Sum
  Anti-windup : Subsystem
  Constant : Constant  Commented=on  Value=Kp_Iab_EMFobs
  Constant2 : Constant  Commented=on  Value=Ki_Iab_EMFobs
  Data Type Conversion : DataTypeConversion  Commented=on
  Ki activation treashold : Constant  Value=0.23  OutDataTypeStr=single
  Kp : Gain  Gain=Kp_Iab_EMFobs  OutDataTypeStr=Inherit: Same as input
  PID Controller : pid_lib/PID Controller  Commented=on  Controller=PI  Form=Parallel  TimeDomain=Discrete-time  UseExternalTs=off  SampleTime=-1  IntegratorMethod=Forward Euler  FilterMethod=Forward Euler  ControllerParametersSource=external  P=1  I=1  D=0  UseFilter=on  N=100  TunerSelectOption=Transfer Function Based (PID Tuner App)  ZeroCross=off  InitialConditionSource=internal  InitialConditionForIntegrator=0  InitialConditionForFilter=0  DifferentiatorICPrevScaledInput=0  ExternalReset=none  TrackingMode=off  Kt=1  LimitOutput=on  SatLimitsSource=internal  UpperSaturationLimit=MaxBckEMFVol_sat_pos  LowerSaturationLimit=MaxBckEMFVol_sat_neg  LinearizeAsGain=on  AntiWindupMode=clamping  Kb=1  POutMin=[]  POutMax=[]  IOutMin=[]  IOutMax=[]  DOutMin=[]  DOutMax=[]  NOutMin=[]  NOutMax=[]  SumOutMin=[]  SumOutMax=[]  SaturationOutMin=[]  SaturationOutMax=[]  PParamMin=[]  PParamMax=[]  IParamMin=[]  IParamMax=[]  DParamMin=[]  DParamMax=[]  NParamMin=[]  NParamMax=[]  KbParamMin=[]  KbParamMax=[]  KtParamMin=[]  KtParamMax=[]  KbOutMin=[]  KbOutMax=[]  KtOutMin=[]  KtOutMax=[]  IntegratorOutMin=[]  IntegratorOutMax=[]  FilterOutMin=[]  FilterOutMax=[]  SumI1OutMin=[]  SumI1OutMax=[]  SumI2OutMin=[]  SumI2OutMax=[]  SumI3OutMin=[]  SumI3OutMax=[]  SumI4OutMin=[]  SumI4OutMax=[]  SumDOutMin=[]  SumDOutMax=[]  DifferentiatorOutMin=[]  DifferentiatorOutMax=[]  FilterDiffOutCoefMin=[]  FilterDiffOutCoefMax=[]  ReciprocalOutMin=[]  ReciprocalOutMax=[]  SumDenOutMin=[]  SumDenOutMax=[]  SumNumOutMin=[]  SumNumOutMax=[]  DivideOutMin=[]  DivideOutMax=[]  UdiffTsProdOutMin=[]  UdiffTsProdOutMax=[]  NTsProdOutMin=[]  NTsProdOutMax=[]  UintegralTsProdOutMin=[]  UintegralTsProdOutMax=[]  UngainTsProdOutMin=[]  UngainTsProdOutMax=[]  IntegratorContinuousStateAttributes=''  IntegratorStateMustResolveToSignalObject=off  IntegratorRTWStateStorageClass=Auto  FilterContinuousStateAttributes=''  FilterStateMustResolveToSignalObject=off  FilterRTWStateStorageClass=Auto  ParallelPVariant=ExternalParameters  IdealPVariant=Disabled  IVariant=ExternalParameters  DVariant=Disabled  IntegratorVariant=Discrete  SatVariant=Enabled  AWVariant=DiscClampingParallel  PCopyVariant=Disabled  TRVariant=Disabled  FdbkBlocksVariant=Forward  IdealPFdbkVariant=Disabled  SatFdbkVariant=Disabled  DerivativeFilterVariant=Disabled  NVariant=Disabled  NCopyVariant=Disabled_SignalSpec  FilterICVariant=Disabled  IntegratorICVariant=InternalICs  ExternalResetVariant=Disabled  TRSumVariant=Passthrough  SumFdbkVariant=Disabled  SumVariant=Sum_PI  TsampFilterVariant=InternalTs  TsampNgainVariant=Passthrough  TsampIntegralVariant=Passthrough  ExternalSaturationOutDataTypeStr=Inherit: Same as second input
  Relational Operator : RelationalOperator  Operator=<=  OutDataTypeStr=boolean  RndMeth=Simplest
  Saturation : Saturate  UpperLimit=MaxBckEMFVol_sat_pos  LowerLimit=MaxBckEMFVol_sat_neg
  Sig_Emfobs_PI_out : Outport
  wires:
  PID Controller/1 -> Data Type Conversion/1
  Kp/1 -> Add1/1
  Anti-windup/1(Out1) -> Add1/2
  Ki activation treashold/1 -> Relational Operator/2
  Add1/1 -> Saturation/1
  Relational Operator/1 -> Anti-windup/Enable
  Constant/1 -> PID Controller/2
  Constant2/1 -> PID Controller/3
  Data Type Conversion/1 -> ?
  Sig_Emfobs_errorSum_m/1 -> PID Controller/1, Anti-windup/1(In1), Abs/1, Kp/1
  Saturation/1 -> Sig_Emfobs_PI_out/1  "Sig_Emfobs_PI_out"
  Abs/1 -> Relational Operator/1
  reset/1 -> Anti-windup/2(In2)

== system MotorControlLibNEWFixedP_FULL19b/Position observer/EMF Observer Ia1/DC Motor Model ==
  note: Integrator
  note: d/dt(i)
  note: i
  In1 : Inport
  In2 : Inport  Port=2
  Add5 : Sum  Inputs=-+-  OutDataTypeStr=Inherit: Same as first input
  Delay : Delay  DelayLength=1  InitialCondition=0
  Gain : Gain  Gain=TsIntern  ParamDataTypeStr=Inherit: Inherit from 'Gain'  OutDataTypeStr=Inherit: Inherit via back propagation
  Inductance : Gain  Gain=Ld  OutDataTypeStr=Inherit: Same as input
  Resistance : Gain  Gain=Rs  OutDataTypeStr=Inherit: Inherit via back propagation
  Sum : Sum  Inputs=|++  OutDataTypeStr=Inherit: Same as first input
  Unit Delay : UnitDelay  SampleTime=-1  HasFrameUpgradeWarning=on
  Out1 : Outport
  wires:
  Gain/1 -> Sum/1
  Delay/1 -> Sum/2
  Inductance/1 -> Gain/1
  Sum/1 -> Resistance/1, Out1/1, Delay/1
  Resistance/1 -> Add5/1
  Unit Delay/1 -> Inductance/1
  In1/1 -> Add5/3
  Add5/1 -> Unit Delay/1
  In2/1 -> Add5/2

== system MotorControlLibNEWFixedP_FULL19b/Position observer/EMF Observer Ia1/PI Controller ==
  In1 : Inport
  In2 : Inport  Port=2
  Add1 : Sum
  Add6 : Sum  Inputs=-+  InputSameDT=on
  Anti-windup : Subsystem
  Constant1 : Constant  Value=0.8  OutDataTypeStr=fixdt(1,32,2^-8,0)
  Kp : Gain  Gain=Kp_Iab_EMFobs  OutDataTypeStr=Inherit: Same as input
  Relational Operator : RelationalOperator  Operator=<=  OutDataTypeStr=boolean  RndMeth=Simplest
  Saturation : Saturate  UpperLimit=MaxBckEMFVol_sat_pos  LowerLimit=MaxBckEMFVol_sat_neg
  Out1 : Outport
  wires:
  In2/1 -> Add6/2
  Add6/1 -> Anti-windup/1(In1), Relational Operator/1, Kp/1
  Anti-windup/1(Out1) -> Add1/2
  Constant1/1 -> Relational Operator/2
  In1/1 -> Add6/1
  Relational Operator/1 -> Anti-windup/Enable
  Add1/1 -> Saturation/1
  Kp/1 -> Add1/1
  Saturation/1 -> Out1/1

== system MotorControlLibNEWFixedP_FULL19b/Position observer/EMF Observer Ia2/DC Motor Model ==
  note: Integrator
  note: d/dt(i)
  note: i
  Sig_Emfobs_PI_out : Inport
  In2 : Inport  Port=2
  Sig_Emfobs_PI_out1 : Inport  Port=3
  Add5 : Sum  Inputs=-+--  OutDataTypeStr=Inherit: Same as first input
  Delay : Delay  DelayLength=1  InitialCondition=0
  Gain : Gain  Gain=TsIntern  ParamDataTypeStr=Inherit: Inherit from 'Gain'  OutMin=-100  OutMax=+100  OutDataTypeStr=fixdt(1,16,2^-4,0)  SaturateOnIntegerOverflow=on
  Inductance : Gain  Gain=Ld  OutDataTypeStr=fixdt(1,16,2^9,0)
  Resistance : Gain  Gain=Rs  OutDataTypeStr=Inherit: Inherit via back propagation
  Sum : Sum  Inputs=|++  OutDataTypeStr=Inherit: Same as first input
  Unit Delay : UnitDelay  SampleTime=-1  HasFrameUpgradeWarning=on
  i_integrated_en8 : Outport
  wires:
  Sum/1 -> Resistance/1, i_integrated_en8/1, Delay/1
  Inductance/1 -> Gain/1
  Add5/1 -> Unit Delay/1
  Sig_Emfobs_PI_out/1 -> Add5/3
  Delay/1 -> Sum/2
  Resistance/1 -> Add5/1
  In2/1 -> Add5/2
  Gain/1 -> Sum/1
  Unit Delay/1 -> Inductance/1
  Sig_Emfobs_PI_out1/1 -> Add5/4

== system MotorControlLibNEWFixedP_FULL19b/Position observer/EMF Observer Ia2/PI Controller ==
  Sig_Emfobs_errorSum_m : Inport
  reset : Inport  Port=2
  Abs : Abs
  Add1 : Sum
  Anti-windup : Subsystem
  Constant : Constant  Commented=on  Value=Kp_Iab_EMFobs
  Constant1 : Constant  Value=0.23  OutDataTypeStr=fixdt(1,16,2^-8,0)
  Constant2 : Constant  Commented=on  Value=Ki_Iab_EMFobs
  Data Type Conversion : DataTypeConversion  Commented=on
  Kp : Gain  Gain=Kp_Iab_EMFobs  ParamDataTypeStr=Inherit: Inherit from 'Gain'  OutDataTypeStr=Inherit: Same as input
  PID Controller : pid_lib/PID Controller  Commented=on  Controller=PI  Form=Parallel  TimeDomain=Discrete-time  UseExternalTs=off  SampleTime=-1  IntegratorMethod=Forward Euler  FilterMethod=Forward Euler  ControllerParametersSource=external  P=1  I=1  D=0  UseFilter=on  N=100  TunerSelectOption=Transfer Function Based (PID Tuner App)  ZeroCross=off  InitialConditionSource=internal  InitialConditionForIntegrator=0  InitialConditionForFilter=0  DifferentiatorICPrevScaledInput=0  ExternalReset=none  TrackingMode=off  Kt=1  LimitOutput=on  SatLimitsSource=internal  UpperSaturationLimit=MaxBckEMFVol_sat_pos  LowerSaturationLimit=MaxBckEMFVol_sat_neg  LinearizeAsGain=on  AntiWindupMode=clamping  Kb=1  POutMin=[]  POutMax=[]  IOutMin=[]  IOutMax=[]  DOutMin=[]  DOutMax=[]  NOutMin=[]  NOutMax=[]  SumOutMin=[]  SumOutMax=[]  SaturationOutMin=[]  SaturationOutMax=[]  PParamMin=[]  PParamMax=[]  IParamMin=[]  IParamMax=[]  DParamMin=[]  DParamMax=[]  NParamMin=[]  NParamMax=[]  KbParamMin=[]  KbParamMax=[]  KtParamMin=[]  KtParamMax=[]  KbOutMin=[]  KbOutMax=[]  KtOutMin=[]  KtOutMax=[]  IntegratorOutMin=[]  IntegratorOutMax=[]  FilterOutMin=[]  FilterOutMax=[]  SumI1OutMin=[]  SumI1OutMax=[]  SumI2OutMin=[]  SumI2OutMax=[]  SumI3OutMin=[]  SumI3OutMax=[]  SumI4OutMin=[]  SumI4OutMax=[]  SumDOutMin=[]  SumDOutMax=[]  DifferentiatorOutMin=[]  DifferentiatorOutMax=[]  FilterDiffOutCoefMin=[]  FilterDiffOutCoefMax=[]  ReciprocalOutMin=[]  ReciprocalOutMax=[]  SumDenOutMin=[]  SumDenOutMax=[]  SumNumOutMin=[]  SumNumOutMax=[]  DivideOutMin=[]  DivideOutMax=[]  UdiffTsProdOutMin=[]  UdiffTsProdOutMax=[]  NTsProdOutMin=[]  NTsProdOutMax=[]  UintegralTsProdOutMin=[]  UintegralTsProdOutMax=[]  UngainTsProdOutMin=[]  UngainTsProdOutMax=[]  IntegratorContinuousStateAttributes=''  IntegratorStateMustResolveToSignalObject=off  IntegratorRTWStateStorageClass=Auto  FilterContinuousStateAttributes=''  FilterStateMustResolveToSignalObject=off  FilterRTWStateStorageClass=Auto  ParallelPVariant=ExternalParameters  IdealPVariant=Disabled  IVariant=ExternalParameters  DVariant=Disabled  IntegratorVariant=Discrete  SatVariant=Enabled  AWVariant=DiscClampingParallel  PCopyVariant=Disabled  TRVariant=Disabled  FdbkBlocksVariant=Forward  IdealPFdbkVariant=Disabled  SatFdbkVariant=Disabled  DerivativeFilterVariant=Disabled  NVariant=Disabled  NCopyVariant=Disabled_SignalSpec  FilterICVariant=Disabled  IntegratorICVariant=InternalICs  ExternalResetVariant=Disabled  TRSumVariant=Passthrough  SumFdbkVariant=Disabled  SumVariant=Sum_PI  TsampFilterVariant=InternalTs  TsampNgainVariant=Passthrough  TsampIntegralVariant=Passthrough  ExternalSaturationOutDataTypeStr=Inherit: Same as second input
  Relational Operator : RelationalOperator  Operator=<=  OutDataTypeStr=boolean  RndMeth=Simplest
  Saturation : Saturate  UpperLimit=MaxBckEMFVol_sat_pos  LowerLimit=MaxBckEMFVol_sat_neg
  Sig_Emfobs_PI_out : Outport
  wires:
  Saturation/1 -> Sig_Emfobs_PI_out/1
  Sig_Emfobs_errorSum_m/1 -> Kp/1, Anti-windup/1(In1), Abs/1, PID Controller/1
  Data Type Conversion/1 -> ?
  Constant2/1 -> PID Controller/3
  Constant/1 -> PID Controller/2
  Relational Operator/1 -> Anti-windup/Enable
  Add1/1 -> Saturation/1
  Constant1/1 -> Relational Operator/2
  Anti-windup/1(Out1) -> Add1/2
  Kp/1 -> Add1/1
  PID Controller/1 -> Data Type Conversion/1
  Abs/1 -> Relational Operator/1
  reset/1 -> Anti-windup/2(In2)

== system MotorControlLibNEWFixedP_FULL19b/Position observer fixed point/EMF Observer Ia/DC Motor Model ==
  note: d/dt(i)
  note: Integrator
  Sig_Emfobs_PI_out : Inport
  In2 : Inport  Port=2
  In3 : Inport  Port=3
  Add5 : Sum  Inputs=-+--  OutDataTypeStr=Inherit: Same as first input
  Data Type Conversion : DataTypeConversion
  Delay : Delay  DelayLength=1  InitialCondition=0  StateName=UnitDelayIntegratorPosObs
  Gain : Gain  Gain=TsIntern  ParamDataTypeStr=Inherit: Inherit from 'Gain'  OutMin=-100  OutMax=+100  OutDataTypeStr=fixdt(1,16,2^-4,0)  SaturateOnIntegerOverflow=on
  Inductance : Gain  Gain=Ld  OutDataTypeStr=fixdt(1,16,2^9,0)
  Resistance : Gain  Gain=Rs  OutDataTypeStr=Inherit: Inherit via back propagation
  Sum : Sum  Inputs=|++  OutDataTypeStr=Inherit: Same as first input
  Unit Delay : UnitDelay  SampleTime=-1  HasFrameUpgradeWarning=on
  i_integrated_en8 : Outport
  wires:
  Unit Delay/1 -> Inductance/1
  Gain/1 -> Sum/1  "di_dt_times_Ts_En8"
  Sum/1 -> Delay/1, Data Type Conversion/1, Resistance/1  "i_integrated_en4"
  In2/1 -> Add5/2
  Resistance/1 -> Add5/1  "i_integrated_times_Rs_en8"
  Delay/1 -> Sum/2
  Sig_Emfobs_PI_out/1 -> Add5/3
  Add5/1 -> Unit Delay/1  "Va_all_16En4"
  Inductance/1 -> Gain/1  "di_dt_E9"
  Data Type Conversion/1 -> i_integrated_en8/1
  In3/1 -> Add5/4

== system MotorControlLibNEWFixedP_FULL19b/Position observer fixed point/EMF Observer Ia/PI Controller ==
  Sig_Emfobs_errorSum_m : Inport
  reset : Inport  Port=2
  Abs : Abs
  Add1 : Sum
  Anti-windup : Subsystem
  Constant : Constant  Commented=on  Value=Kp_Iab_EMFobs
  Constant2 : Constant  Commented=on  Value=Ki_Iab_EMFobs
  Data Type Conversion : DataTypeConversion  Commented=on
  Ki activation treashold : Constant  Value=0.23  OutDataTypeStr=fixdt(1,16,2^-8,0)
  Kp : Gain  Gain=Kp_Iab_EMFobs  OutDataTypeStr=Inherit: Same as input
  PID Controller : pid_lib/PID Controller  Commented=on  Controller=PI  Form=Parallel  TimeDomain=Discrete-time  UseExternalTs=off  SampleTime=-1  IntegratorMethod=Forward Euler  FilterMethod=Forward Euler  ControllerParametersSource=external  P=1  I=1  D=0  UseFilter=on  N=100  TunerSelectOption=Transfer Function Based (PID Tuner App)  ZeroCross=off  InitialConditionSource=internal  InitialConditionForIntegrator=0  InitialConditionForFilter=0  DifferentiatorICPrevScaledInput=0  ExternalReset=none  TrackingMode=off  Kt=1  LimitOutput=on  SatLimitsSource=internal  UpperSaturationLimit=MaxBckEMFVol_sat_pos  LowerSaturationLimit=MaxBckEMFVol_sat_neg  LinearizeAsGain=on  AntiWindupMode=clamping  Kb=1  POutMin=[]  POutMax=[]  IOutMin=[]  IOutMax=[]  DOutMin=[]  DOutMax=[]  NOutMin=[]  NOutMax=[]  SumOutMin=[]  SumOutMax=[]  SaturationOutMin=[]  SaturationOutMax=[]  PParamMin=[]  PParamMax=[]  IParamMin=[]  IParamMax=[]  DParamMin=[]  DParamMax=[]  NParamMin=[]  NParamMax=[]  KbParamMin=[]  KbParamMax=[]  KtParamMin=[]  KtParamMax=[]  KbOutMin=[]  KbOutMax=[]  KtOutMin=[]  KtOutMax=[]  IntegratorOutMin=[]  IntegratorOutMax=[]  FilterOutMin=[]  FilterOutMax=[]  SumI1OutMin=[]  SumI1OutMax=[]  SumI2OutMin=[]  SumI2OutMax=[]  SumI3OutMin=[]  SumI3OutMax=[]  SumI4OutMin=[]  SumI4OutMax=[]  SumDOutMin=[]  SumDOutMax=[]  DifferentiatorOutMin=[]  DifferentiatorOutMax=[]  FilterDiffOutCoefMin=[]  FilterDiffOutCoefMax=[]  ReciprocalOutMin=[]  ReciprocalOutMax=[]  SumDenOutMin=[]  SumDenOutMax=[]  SumNumOutMin=[]  SumNumOutMax=[]  DivideOutMin=[]  DivideOutMax=[]  UdiffTsProdOutMin=[]  UdiffTsProdOutMax=[]  NTsProdOutMin=[]  NTsProdOutMax=[]  UintegralTsProdOutMin=[]  UintegralTsProdOutMax=[]  UngainTsProdOutMin=[]  UngainTsProdOutMax=[]  IntegratorContinuousStateAttributes=''  IntegratorStateMustResolveToSignalObject=off  IntegratorRTWStateStorageClass=Auto  FilterContinuousStateAttributes=''  FilterStateMustResolveToSignalObject=off  FilterRTWStateStorageClass=Auto  ParallelPVariant=ExternalParameters  IdealPVariant=Disabled  IVariant=ExternalParameters  DVariant=Disabled  IntegratorVariant=Discrete  SatVariant=Enabled  AWVariant=DiscClampingParallel  PCopyVariant=Disabled  TRVariant=Disabled  FdbkBlocksVariant=Forward  IdealPFdbkVariant=Disabled  SatFdbkVariant=Disabled  DerivativeFilterVariant=Disabled  NVariant=Disabled  NCopyVariant=Disabled_SignalSpec  FilterICVariant=Disabled  IntegratorICVariant=InternalICs  ExternalResetVariant=Disabled  TRSumVariant=Passthrough  SumFdbkVariant=Disabled  SumVariant=Sum_PI  TsampFilterVariant=InternalTs  TsampNgainVariant=Passthrough  TsampIntegralVariant=Passthrough  ExternalSaturationOutDataTypeStr=Inherit: Same as second input
  Relational Operator : RelationalOperator  Operator=<=  OutDataTypeStr=boolean  RndMeth=Simplest
  Saturation : Saturate  UpperLimit=MaxBckEMFVol_sat_pos  LowerLimit=MaxBckEMFVol_sat_neg
  Sig_Emfobs_PI_out : Outport
  wires:
  PID Controller/1 -> Data Type Conversion/1
  Kp/1 -> Add1/1
  Anti-windup/1(Out1) -> Add1/2
  Ki activation treashold/1 -> Relational Operator/2
  Add1/1 -> Saturation/1
  Relational Operator/1 -> Anti-windup/Enable
  Constant/1 -> PID Controller/2
  Constant2/1 -> PID Controller/3
  Data Type Conversion/1 -> ?
  Sig_Emfobs_errorSum_m/1 -> PID Controller/1, Anti-windup/1(In1), Abs/1, Kp/1
  Saturation/1 -> Sig_Emfobs_PI_out/1  "Sig_Emfobs_PI_out"
  Abs/1 -> Relational Operator/1
  reset/1 -> Anti-windup/2(In2)
